simulink model "DMARC"  (R2018a)
settings: Solver=ode45  StartTime=0.0  StopTime=10  RelTol=1e-3  EnableMultiTasking=on
InitFcn:
  | u = 0;
  | ym = 0;
  | y = 0.5;
  | eo = 0;
  | am = 1;
  | km = 1;
  | ap = -1;
  | kp = 1;
  | theta1 = 0;
  | theta2 = 0;
  | theta1_estimated = 2.1;
  | theta2_estimated = 1.1;
  | sigma = 1;
  | L = 1000000;
  | mi = 0;
settings Model: Creator=danilopena  LastModifiedBy=LIME
settings DataIOCC: LimitDataPoints=on  SaveFormat=Array
settings OptimizationCC: LifeSpan=inf
settings DebuggingCC: UnderspecifiedInitializationDetection=Classic  MergeDetectMultiDrivingBlocksExec=none  SolverPrmCheckMsg=warning  StateNameClashWarn=warning  SFUnexpectedBacktrackingDiag=warning  SFNoUnconditionalDefaultTransitionDiag=warning  SFExecutionAtInitializationDiag=none
settings HardwareCC: ProdBitPerPointer=32  ProdBitPerSizeT=32  ProdBitPerPtrDiffT=32  ProdLargestAtomicFloat=None  ProdIntDivRoundTo=Undefined  ProdEndianess=Unspecified  ProdWordSize=32  ProdHWDeviceType=32-bit Generic
settings ModelReferenceCC: PropagateSignalLabelsOutOfModel=off
settings CodeAppCC: StateflowObjectComments=on
settings GRTTargetCC: TargetLangStandard=C89/C90 (ANSI)  GeneratePreprocessorConditionals=Disable all
settings ConfigComp: CovMetricSettings=dw  CovHtmlReporting=on  CovSaveCumulativeToWorkspaceVar=on  CovSaveSingleToWorkspaceVar=on  CovExternalEMLEnable=off

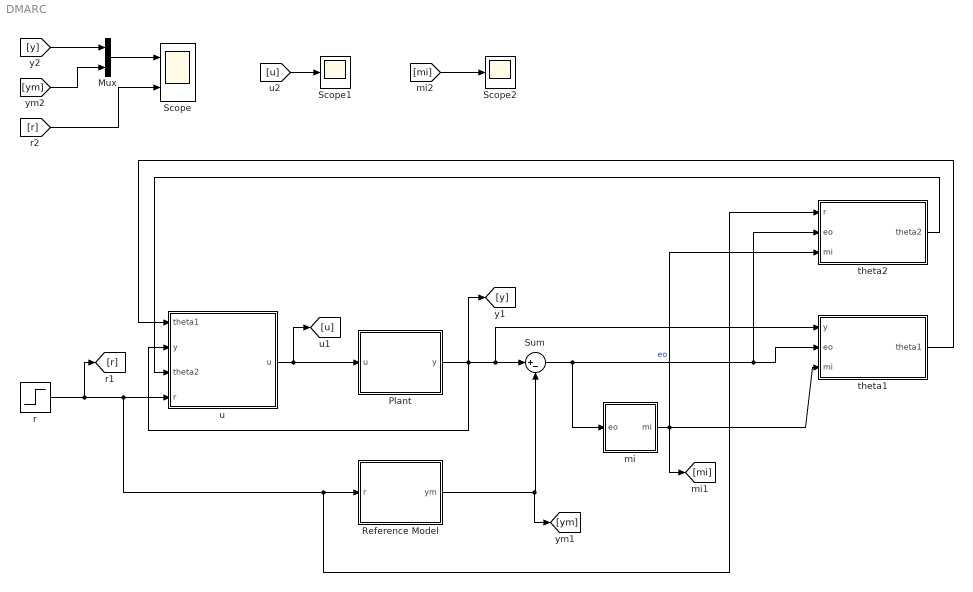
== system DMARC ==
  Mux : Mux  Inputs=2
  Plant : Subsystem
  Reference Model : Subsystem
  Scope : Scope  NumInputPorts=2
  Scope1 : Scope
  Scope2 : Scope
  Sum : Sum  Inputs=|+-
  mi : Subsystem
  r : Step  SampleTime=0
  theta1 : Subsystem
  theta2 : Subsystem
  u : Subsystem
  wires:
  Plant/1(y) -> [y], u/2(y), theta1/1(y), Sum/1
  Reference Model/1(ym) -> [ym], Sum/2
  Sum/1 -> theta2/2(eo), theta1/2(eo), mi/1(eo)  "eo"
  u/1(u) -> [u], Plant/1(u)
  r/1 -> [r], theta2/1(r), Reference Model/1(r), u/4(r)
  [r] -> Scope/2
  [y] -> Mux/1
  [ym] -> Mux/2
  Mux/1 -> Scope/1
  mi/1(mi) -> theta2/3(mi), theta1/3(mi), [mi]
  [u] -> Scope1/1
  [mi] -> Scope2/1
  theta2/1(theta2) -> u/3(theta2)
  theta1/1(theta1) -> u/1(theta1)

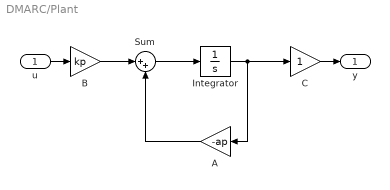
== system DMARC/Plant ==
  u : Inport
  A : Gain  Gain=-ap
  B : Gain  Gain=kp
  C : Gain
  Integrator : Integrator
  Sum : Sum  Inputs=|++
  y : Outport
  wires:
  B/1 -> Sum/1
  A/1 -> Sum/2
  Sum/1 -> Integrator/1
  Integrator/1 -> C/1, A/1
  u/1 -> B/1
  C/1 -> y/1

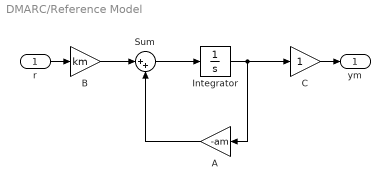
== system DMARC/Reference Model ==
  r : Inport
  A : Gain  Gain=-am
  B : Gain  Gain=km
  C : Gain
  Integrator : Integrator
  Sum : Sum  Inputs=|++
  ym : Outport
  wires:
  B/1 -> Sum/1
  A/1 -> Sum/2
  Sum/1 -> Integrator/1
  Integrator/1 -> C/1, A/1
  r/1 -> B/1
  C/1 -> ym/1

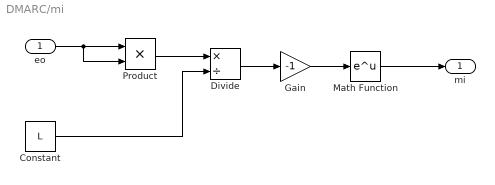
== system DMARC/mi ==
  eo : Inport
  Constant : Constant  Value=L
  Divide : Product  Inputs=*/
  Gain : Gain  Gain=-1
  Math Function : Math  SaturateOnIntegerOverflow=on
  Product : Product
  mi : Outport
  wires:
  eo/1 -> Product/2, Product/1
  Product/1 -> Divide/1
  Constant/1 -> Divide/2
  Divide/1 -> Gain/1
  Gain/1 -> Math Function/1
  Math Function/1 -> mi/1

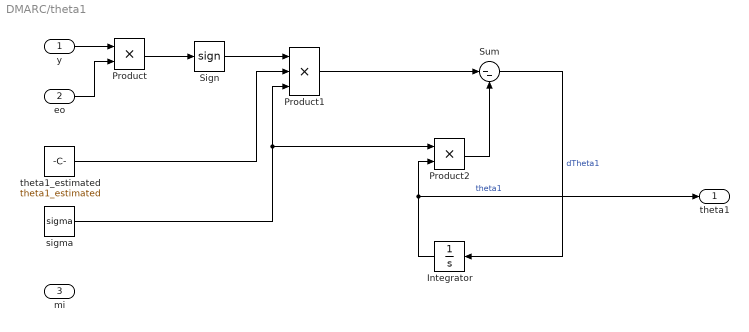
== system DMARC/theta1 ==
  y : Inport
  eo : Inport  Port=2
  mi : Inport  Port=3
  Integrator : Integrator
  Product : Product
  Product1 : Product  Inputs=3
  Product2 : Product
  Sign : Signum
  Sum : Sum  Inputs=|--
  sigma : Constant  Value=sigma
  theta1_estimated : Constant  Value=theta1_estimated
  theta1 : Outport
  wires:
  y/1 -> Product/1
  eo/1 -> Product/2
  Product/1 -> Sign/1
  Sign/1 -> Product1/1
  theta1_estimated/1 -> Product1/2
  sigma/1 -> Product2/1, Product1/3
  Product2/1 -> Sum/2
  Product1/1 -> Sum/1
  Sum/1 -> Integrator/1  "dTheta1"
  Integrator/1 -> Product2/2, theta1/1  "theta1"

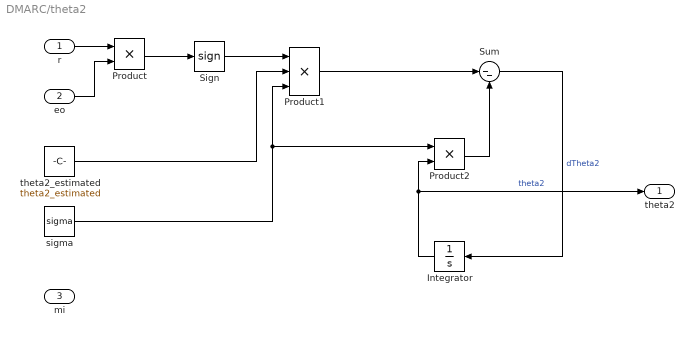
== system DMARC/theta2 ==
  r : Inport
  eo : Inport  Port=2
  mi : Inport  Port=3
  Integrator : Integrator
  Product : Product
  Product1 : Product  Inputs=3
  Product2 : Product
  Sign : Signum
  Sum : Sum  Inputs=|--
  sigma : Constant  Value=sigma
  theta2_estimated : Constant  Value=theta2_estimated
  theta2 : Outport
  wires:
  r/1 -> Product/1
  eo/1 -> Product/2
  Product/1 -> Sign/1
  Sign/1 -> Product1/1
  theta2_estimated/1 -> Product1/2
  sigma/1 -> Product2/1, Product1/3
  Product2/1 -> Sum/2
  Product1/1 -> Sum/1
  Sum/1 -> Integrator/1  "dTheta2"
  Integrator/1 -> theta2/1, Product2/2  "theta2"

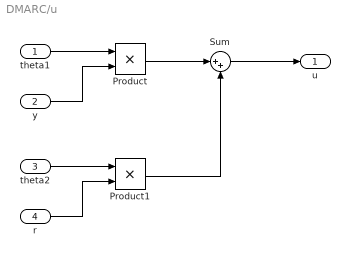
== system DMARC/u ==
  theta1 : Inport
  y : Inport  Port=2
  theta2 : Inport  Port=3
  r : Inport  Port=4
  Product : Product
  Product1 : Product
  Sum : Sum  Inputs=|++
  u : Outport
  wires:
  y/1 -> Product/2
  theta1/1 -> Product/1
  r/1 -> Product1/2
  theta2/1 -> Product1/1
  Product/1 -> Sum/1
  Product1/1 -> Sum/2
  Sum/1 -> u/1
